simulink model "Ather_450x"  (R2024a)
settings: Solver=VariableStepAuto  StartTime=0.0  StopTime=inf  MaxStep=0.001  RelTol=1e-3
undefined symbols (not defined in the file): magnitude
libraries: simulink_extras x1
settings Model: Creator=appu  LastModifiedBy=appu

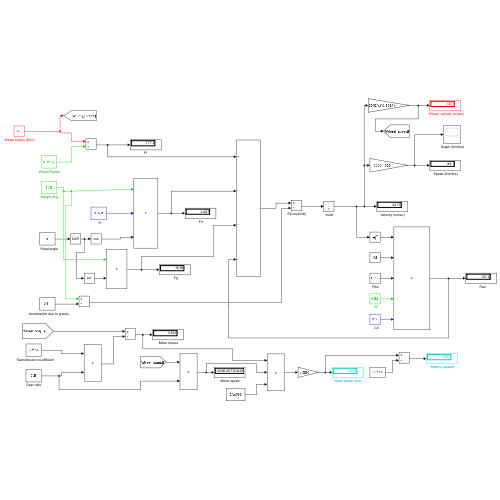
[thumbnail: Simulink's stored preview of the top-level diagram]
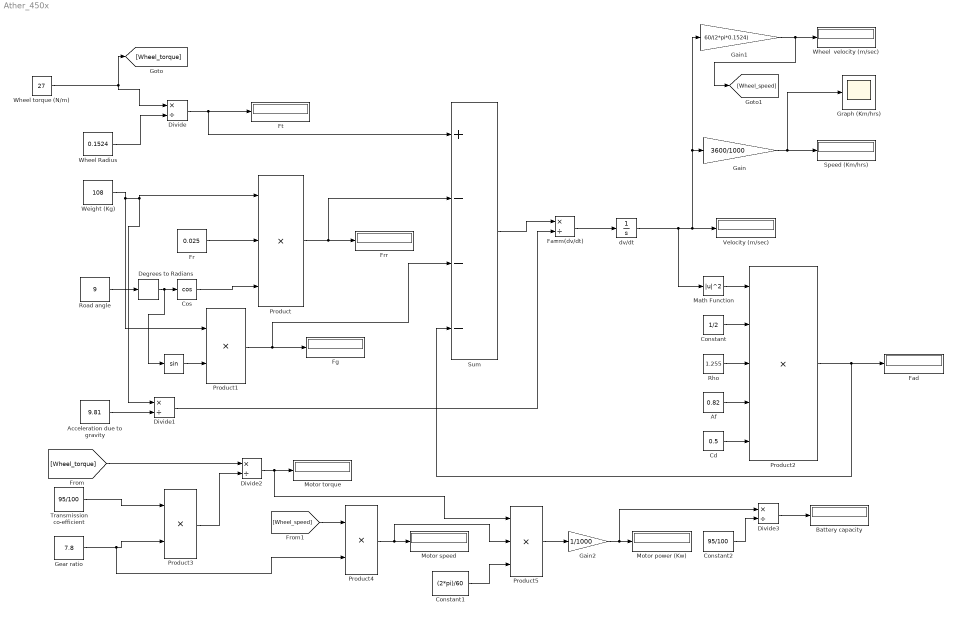
== system Ather_450x ==
  " " : Trigonometry
  "      Gear ratio      " : Constant  Value=7.8
  "    Road angle" : Constant  Value=9
  "   Acceleration due to gravity" : Constant  Value=9.81
  "   Cd" : Constant  Value=0.5
  "   Fad" : Display
  "   Fr" : Constant  Value=0.025
  "   Transmission co-efficient" : Constant  Value=95/100
  "   Wheel  velocity (m/sec)" : Display
  "  Af" : Constant  Value=0.82
  "  Battery capacity" : Display
  "  Fg" : Display
  " Fa=m(dv/dt)" : Product  Inputs=*/
  " Frr" : Display
  " Graph (Km/hrs)" : Scope
  " Motor power (Kw)" : Display
  " Motor speed" : Display
  " Motor torque" : Display
  " Rho" : Constant  Value=1.255
  " Speed (Km/hrs)" : Display
  " Velocity (m/sec)" : Display
  " Weight (Kg)" : Constant  Value=108
  " Wheel Radius" : Constant  Value=0.1524
  " Wheel torque (N/m)" : Constant  Value=27
  " dv/dt" : Integrator
  Constant : Constant  Value=1/2
  Constant1 : Constant  Value=(2*pi)/60
  Constant2 : Constant  Value=95/100
  Cos : Trigonometry  Operator=cos
  Degrees to Radians : simulink_extras/Transformations/Degrees to Radians
  Divide{,1..3} (4 alike) : Product  Inputs=*/
  Ft : Display
  Gain : Gain  Gain=3600/1000
  Gain1 : Gain  Gain=60/(2*pi*0.1524)
  Gain2 : Gain  Gain=1/1000
  Math Function : Math  Operator=magnitude^2
  Product : Product  Inputs=3
  Product1 : Product
  Product2 : Product  Inputs=5
  Product3 : Product
  Product4 : Product
  Product5 : Product  Inputs=3
  Sum : Sum  Inputs=+---
  wires:
  " Wheel Radius"/1 -> Divide/2
  Divide/1 -> Sum/1, Ft/1
  "    Road angle"/1 -> Degrees to Radians/1
  Degrees to Radians/1 -> " "/1, Cos/1
  " Weight (Kg)"/1 -> Product1/1, Divide1/1, Product/1
  "   Fr"/1 -> Product/2
  Cos/1 -> Product/3
  Product/1 -> Sum/2, " Frr"/1
  " "/1 -> Product1/2
  Product1/1 -> Sum/3, "  Fg"/1
  "   Acceleration due to gravity"/1 -> Divide1/2
  " Fa=m(dv/dt)"/1 -> " dv/dt"/1
  " dv/dt"/1 -> Math Function/1, Gain1/1, Gain/1, " Velocity (m/sec)"/1
  Math Function/1 -> Product2/1
  Constant/1 -> Product2/2
  " Rho"/1 -> Product2/3
  "  Af"/1 -> Product2/4
  "   Cd"/1 -> Product2/5
  Product2/1 -> Sum/4, "   Fad"/1
  Gain/1 -> " Graph (Km/hrs)"/1, " Speed (Km/hrs)"/1
  Gain1/1 -> [Wheel_speed], "   Wheel  velocity (m/sec)"/1
  "   Transmission co-efficient"/1 -> Product3/1
  "      Gear ratio      "/1 -> Product4/2, Product3/2
  [Wheel_torque] -> Divide2/1
  Product3/1 -> Divide2/2
  Divide2/1 -> Product5/1, " Motor torque"/1
  [Wheel_speed] -> Product4/1
  Product4/1 -> Product5/2, " Motor speed"/1
  Constant1/1 -> Product5/3
  Product5/1 -> Gain2/1
  Gain2/1 -> Divide3/1, " Motor power (Kw)"/1
  Constant2/1 -> Divide3/2
  Divide3/1 -> "  Battery capacity"/1
  " Wheel torque (N/m)"/1 -> Divide/1, [Wheel_torque]
  Sum/1 -> " Fa=m(dv/dt)"/1
  Divide1/1 -> " Fa=m(dv/dt)"/2
